simulink model "buttonblink_task"  (Simulink 3.00)
libraries: genlib x2, mathlib x2, logiclib x1

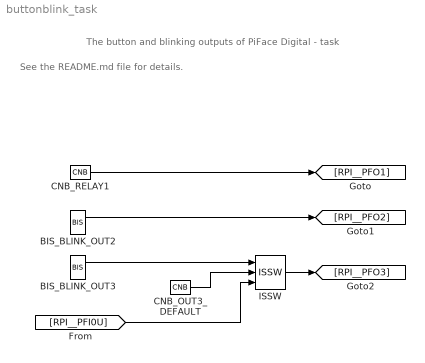
== system buttonblink_task ==
  note: See the README.md file for details.
  note: The button and blinking outputs of PiFace Digital - task
  BIS_BLINK_OUT2 : genlib/BIS  Y0=off  t1=1  t2=2  t3=0  t4=4  t5=5  t6=6  t7=7  t8=8  RPT=on  bEdit=off
  BIS_BLINK_OUT3 : genlib/BIS  Y0=off  t1=0.2  t2=0.4  t3=0  t4=0  t5=0  t6=0  t7=2.0  t8=0  RPT=on  bEdit=off
  CNB_OUT3_DEFAULT : mathlib/CNB  YCN=off
  CNB_RELAY1 : mathlib/CNB  YCN=on
  ISSW : logiclib/ISSW
  wires:
  BIS_BLINK_OUT2/1 -> [RPI__PFO2]
  BIS_BLINK_OUT3/1 -> ISSW/1
  CNB_OUT3_DEFAULT/1 -> ISSW/2
  CNB_RELAY1/1 -> [RPI__PFO1]
  [RPI__PFI0U] -> ISSW/3
  ISSW/1 -> [RPI__PFO3]
